simulink model "FlightDataRecorder"  (R2023b)
settings: Solver=VariableStepAuto  StartTime=0.0  StopTime=inf  RelTol=1e-3
libraries: dspindex x28, simulink x4, dspnetwork x4, etargetslib x3, aerolibconvert2 x1
(part 3 of 3)

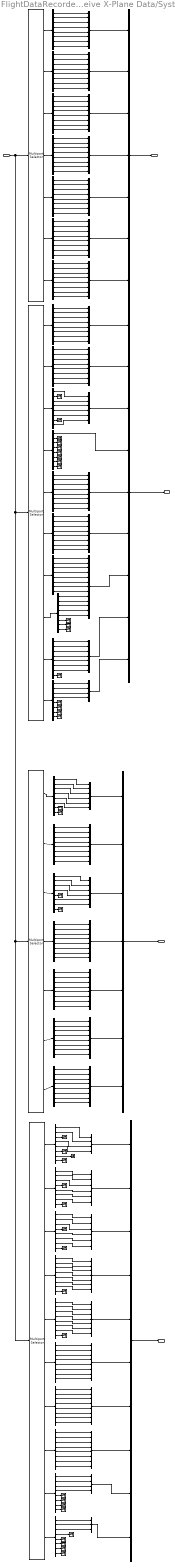
== system FlightDataRecorder/Receive X-Plane Data/Systems ==
  Data : Inport
  Bus Creator{1,3,5..6,11,13..16,18,25..33} (19 alike) : BusCreator  Inputs=8
  Bus Creator{4,10,12,21..22} (5 alike) : BusCreator  Inputs=6
  Bus Creator{8,17,19,23..24} (5 alike) : BusCreator  Inputs=7
  Bus Creator2 : BusCreator  Inputs=9
  Bus Creator20 : BusCreator  Inputs=4
  Bus Creator34 : BusCreator  Inputs=4
  Bus Creator35 : BusCreator  Inputs=3
  Bus Creator36 : BusCreator  Inputs=10
  Bus Creator7 : BusCreator  Inputs=13
  Bus Creator9 : BusCreator  Inputs=4
  Demux{1..34} (34 alike) : Demux  Outputs=8
  Select rows1 : dspindex/Multiport Selector  rowsOrCols=Rows  idxCellArray={107,108,109,110,111,112,113}  idxErrMode=Clip Index
  Select rows2 : dspindex/Multiport Selector  rowsOrCols=Rows  idxCellArray={56,57,58,59,60,61,62}  idxErrMode=Clip Index
  Select rows3 : dspindex/Multiport Selector  rowsOrCols=Rows  idxCellArray={120,121,122,123,124,125,126,127,128,129}  idxErrMode=Clip Index
  Select rows4 : dspindex/Multiport Selector  rowsOrCols=Rows  idxCellArray={97,98,99,100,101,102,103,104,105,106}  idxErrMode=Clip Index
  Terminator{,1..39} (40 alike) : Terminator
  Power systems : Outport
  Operational systems : Outport  Port=2
  Switches : Outport  Port=3
  NAVAID : Outport  Port=4
  wires:
  Demux26/1 -> Bus Creator29/1  "invr 1"
  Bus Creator30/1 -> Bus Creator19/6  "FADEC"
  Demux27/1 -> Bus Creator30/1  "fadec 1"
  Select rows2/6 -> Demux27/1
  Demux27/5 -> Bus Creator30/5  "fadec 5"
  Demux27/3 -> Bus Creator30/3  "fadec 3"
  Demux27/2 -> Bus Creator30/2  "fadec 2"
  Demux27/4 -> Bus Creator30/4  "fadec 4"
  Demux27/6 -> Bus Creator30/6  "fadec 6"
  Demux27/7 -> Bus Creator30/7  "fadec 7"
  Demux27/8 -> Bus Creator30/8  "fadec 8"
  Bus Creator29/1 -> Bus Creator19/5  "Inverter"
  Select rows2/5 -> Demux26/1
  Demux26/5 -> Bus Creator29/5  "invr 5"
  Demux26/3 -> Bus Creator29/3  "invr 3"
  Demux26/2 -> Bus Creator29/2  "invr 2"
  Demux26/4 -> Bus Creator29/4  "invr 4"
  Demux26/6 -> Bus Creator29/6  "invr 6"
  Demux26/7 -> Bus Creator29/7  "invr 7"
  Demux26/8 -> Bus Creator29/8  "invr 8"
  Bus Creator28/1 -> Bus Creator19/4  "Generator"
  Select rows2/4 -> Demux25/1
  Demux25/5 -> Bus Creator28/5  "gen 5"
  Demux25/3 -> Bus Creator28/3  "gen 3"
  Demux25/2 -> Bus Creator28/2  "gen 2"
  Demux25/1 -> Bus Creator28/1  "gen 1"
  Demux25/4 -> Bus Creator28/4  "gen 4"
  Demux25/6 -> Bus Creator28/6  "gen 6"
  Demux25/7 -> Bus Creator28/7  "gen 7"
  Demux25/8 -> Bus Creator28/8  "gen 8"
  Bus Creator27/1 -> Bus Creator19/3  "Battery"
  Select rows2/3 -> Demux24/1
  Demux24/5 -> Bus Creator27/5  "batt 5"
  Demux24/3 -> Bus Creator27/3  "batt 3"
  Demux24/2 -> Bus Creator27/2  "batt 2"
  Demux24/1 -> Bus Creator27/1  "batt 1"
  Demux24/4 -> Bus Creator27/4  "batt 4"
  Demux24/6 -> Bus Creator27/6  "batt 6"
  Demux24/7 -> Bus Creator27/7  "batt 7"
  Demux24/8 -> Bus Creator27/8  "batt 8"
  Demux23/5 -> Bus Creator26/5  "eng idle 5"
  Demux23/3 -> Bus Creator26/3  "eng idle 3"
  Demux23/2 -> Bus Creator26/2  "eng idle 2"
  Demux23/1 -> Bus Creator26/1  "eng idle 1"
  Demux23/4 -> Bus Creator26/4  "eng idle 4"
  Demux23/6 -> Bus Creator26/6  "eng idle 6"
  Bus Creator26/1 -> Bus Creator19/2  "Engine idling"
  Select rows2/2 -> Demux23/1
  Demux23/7 -> Bus Creator26/7  "eng idle 7"
  Demux23/8 -> Bus Creator26/8  "eng idle 8"
  Bus Creator25/1 -> Bus Creator19/1  "Fuel pump"
  Select rows2/1 -> Demux22/1
  Demux22/2 -> Bus Creator25/2  "fuel pump 2"
  Demux22/6 -> Bus Creator25/6  "fuel pump 6"
  Demux22/5 -> Bus Creator25/5  "fuel pump 5"
  Demux22/3 -> Bus Creator25/3  "fuel pump 3"
  Demux22/7 -> Bus Creator25/7  "fuel pump 7"
  Demux22/4 -> Bus Creator25/4  "fuel pump 4"
  Demux22/1 -> Bus Creator25/1  "fuel pump 1"
  Demux22/8 -> Bus Creator25/8  "fuel pump 8"
  Bus Creator18/1 -> Bus Creator19/7  "Ignitier"
  Select rows2/7 -> Demux17/1
  Bus Creator19/1 -> Power systems/1  "Power systems"
  Demux17/2 -> Bus Creator18/2  "igniter 2"
  Demux17/6 -> Bus Creator18/6  "igniter 6"
  Demux17/5 -> Bus Creator18/5  "igniter 5"
  Demux17/3 -> Bus Creator18/3  "igniter 3"
  Demux17/7 -> Bus Creator18/7  "igniter 7"
  Demux17/4 -> Bus Creator18/4  "igniter 4"
  Demux17/1 -> Bus Creator18/1  "igniter 1"
  Demux17/8 -> Bus Creator18/8  "igniter 8"
  Data/1 -> Select rows4/1, Select rows1/1, Select rows3/1, Select rows2/1
  Select rows3/1 -> Demux1/1
  Demux1/2 -> Bus Creator1/2  "pitch"
  Demux1/6 -> Bus Creator1/6  "elevator"
  Demux1/5 -> Bus Creator1/5  "rudder"
  Demux1/3 -> Bus Creator1/3  "R (deg/s)"
  Demux1/7 -> Bus Creator1/7  "speed (knt)"
  Demux1/4 -> Bus Creator1/4  "Q (deg/s)"
  Demux1/1 -> Bus Creator1/1  "heading"
  Demux1/8 -> Bus Creator1/8  "distance (ft)"
  Bus Creator1/1 -> Bus Creator2/1  "Weapon"
  Select rows3/2 -> Demux2/1
  Demux2/2 -> Bus Creator3/2  "vvi cmd"
  Demux2/6 -> Bus Creator3/6  "pressure diff (psi)"
  Demux2/5 -> Bus Creator3/5  "test"
  Demux2/3 -> Bus Creator3/3  "cabin altitude actual"
  Demux2/7 -> Bus Creator3/7  "dump"
  Demux2/4 -> Bus Creator3/4  "vvi actual"
  Demux2/1 -> Bus Creator3/1  "cabin altitude cmd"
  Demux2/8 -> Bus Creator3/8  "bleed"
  Bus Creator3/1 -> Bus Creator2/2  "Pressurisation"
  Select rows3/3 -> Demux3/1
  Demux3/1 -> Bus Creator4/1  "apu equipped"
  Bus Creator4/1 -> Bus Creator2/3  "APU/GPU"
  Demux3/2 -> Terminator/1
  Demux3/3 -> Bus Creator4/2  "apu switch"
  Demux3/4 -> Bus Creator4/3  "apu running"
  Demux3/5 -> Bus Creator4/4  "apu N1"
  Demux3/6 -> Bus Creator4/5  "apu generating"
  Demux3/8 -> Bus Creator4/6  "gpu power"
  Demux3/7 -> Terminator1/1
  Select rows3/4 -> Demux4/1
  Demux4/2 -> Terminator2/1
  Demux4/3 -> Terminator3/1
  Demux4/4 -> Terminator4/1
  Demux4/5 -> Terminator5/1
  Demux4/6 -> Terminator6/1
  Demux4/7 -> Terminator7/1
  Demux4/8 -> Terminator8/1
  Demux4/1 -> Bus Creator2/4  "Radar target"
  Select rows3/5 -> Demux5/1
  Demux5/2 -> Bus Creator5/2  "pump 2a"
  Demux5/6 -> Bus Creator5/6  "fluid 2"
  Demux5/5 -> Bus Creator5/5  "fluid 1"
  Demux5/3 -> Bus Creator5/3  "pump 1b"
  Demux5/7 -> Bus Creator5/7  "pressure 1"
  Demux5/4 -> Bus Creator5/4  "pump 2b"
  Bus Creator5/1 -> Bus Creator2/5  "Hydraulics"
  Demux5/8 -> Bus Creator5/8  "pressure 2"
  Demux5/1 -> Bus Creator5/1  "pump 1a"
  Select rows3/6 -> Demux6/1
  Demux6/2 -> Bus Creator6/2  "bus current 2"
  Demux6/6 -> Bus Creator6/6  "solar output (W)"
  Demux6/5 -> Bus Creator6/5  "eng input (W)"
  Demux6/3 -> Bus Creator6/3  "bus volt 1"
  Demux6/7 -> Bus Creator6/7  "batt capacity (W-hr)"
  Demux6/4 -> Bus Creator6/4  "bus volt 2"
  Demux6/8 -> Bus Creator6/8  "cross"
  Demux6/1 -> Bus Creator6/1  "bus current 1"
  Bus Creator6/1 -> Bus Creator2/6  "Electrical and Solar"
  Select rows3/7 -> Demux7/1
  Demux7/2 -> Bus Creator7/2  "inlet 2"
  Demux7/6 -> Bus Creator7/6  "pitot 2"
  Demux7/5 -> Bus Creator7/5  "pitot 1"
  Demux7/3 -> Bus Creator7/3  "propeller 1"
  Demux7/7 -> Bus Creator7/7  "static 1"
  Demux7/4 -> Bus Creator7/4  "propeller 2"
  Demux7/8 -> Bus Creator7/8  "static 2"
  Demux7/1 -> Bus Creator7/1  "inlet 1"
  Select rows3/8 -> Demux8/1
  Demux8/6 -> Terminator9/1
  Demux8/7 -> Terminator10/1
  Demux8/8 -> Terminator11/1
  Demux8/2 -> Bus Creator7/10  "aoa 2"
  Demux8/5 -> Bus Creator7/13  "window"
  Demux8/3 -> Bus Creator7/11  "left wing"
  Demux8/1 -> Bus Creator7/9  "aoa 1"
  Demux8/4 -> Bus Creator7/12  "right wing"
  Bus Creator7/1 -> Bus Creator2/7  "Icing"
  Select rows3/9 -> Demux9/1
  Demux9/2 -> Bus Creator8/2  "caut time"
  Demux9/6 -> Bus Creator8/6  "gear warning"
  Demux9/5 -> Bus Creator8/5  "gear work"
  Demux9/3 -> Bus Creator8/3  "warning work"
  Demux9/7 -> Bus Creator8/7  "stall warning"
  Demux9/4 -> Bus Creator8/4  "caut work"
  Demux9/1 -> Bus Creator8/1  "warning time"
  Bus Creator8/1 -> Bus Creator2/8  "Warnings"
  Demux9/8 -> Terminator12/1
  Select rows3/10 -> Demux10/1
  Demux10/1 -> Bus Creator9/1  "leg time"
  Demux10/2 -> Bus Creator9/2  "leg type"
  Demux10/3 -> Bus Creator9/3  "leg latitude"
  Demux10/4 -> Bus Creator9/4  "leg longitude"
  Demux10/5 -> Terminator13/1
  Demux10/6 -> Terminator14/1
  Demux10/7 -> Terminator15/1
  Demux10/8 -> Terminator16/1
  Bus Creator9/1 -> Bus Creator2/9  "Flight plan legs"
  Bus Creator2/1 -> Operational systems/1  "Operational systems"
  Select rows1/1 -> Demux11/1
  Demux11/2 -> Bus Creator10/2  "NAV lights"
  Demux11/6 -> Bus Creator10/6  "Taxi lights"
  Demux11/5 -> Bus Creator10/5  "Landing lights"
  Demux11/3 -> Bus Creator10/3  "Beacon lights"
  Demux11/4 -> Bus Creator10/4  "Strobe lights"
  Demux11/1 -> Bus Creator10/1  "AVIO"
  Demux11/8 -> Terminator17/1
  Demux11/7 -> Terminator18/1
  Bus Creator10/1 -> Bus Creator17/1  "Light switches"
  Demux12/2 -> Bus Creator11/2  "EFIS 1"
  Demux12/6 -> Bus Creator11/6  "HSI arc"
  Demux12/5 -> Bus Creator11/5  "HSI 2"
  Demux12/3 -> Bus Creator11/3  "EFIS 2"
  Demux12/4 -> Bus Creator11/4  "HSI 1"
  Demux12/1 -> Bus Creator11/1  "ECAM"
  Demux12/8 -> Bus Creator11/8  "map range"
  Demux12/7 -> Bus Creator11/7  "map"
  Select rows1/2 -> Demux12/1
  Bus Creator11/1 -> Bus Creator17/2  "EFIS"
  Select rows1/3 -> Demux13/1
  Bus Creator12/1 -> Bus Creator17/3  "AP/FDIR/HUD"
  Demux13/5 -> Terminator19/1
  Demux13/8 -> Terminator20/1
  Demux14/2 -> Bus Creator13/2  "inlet"
  Demux14/6 -> Bus Creator13/6  "pitot 2"
  Demux14/5 -> Bus Creator13/5  "pitot 1"
  Demux14/3 -> Bus Creator13/3  "propeller"
  Demux14/4 -> Bus Creator13/4  "windows"
  Demux14/1 -> Bus Creator13/1  "all"
  Demux14/8 -> Bus Creator13/8  "wing"
  Demux14/7 -> Bus Creator13/7  "AOA"
  Select rows1/4 -> Demux14/1
  Bus Creator13/1 -> Bus Creator17/4  "Anti-ice"
  Demux15/2 -> Bus Creator14/2  "air 2"
  Demux15/6 -> Bus Creator14/6  "manual ignition 2"
  Demux15/5 -> Bus Creator14/5  "manual ignition 1"
  Demux15/3 -> Bus Creator14/3  "auto ignition 1"
  Demux15/4 -> Bus Creator14/4  "auto ignition 2"
  Demux15/1 -> Bus Creator14/1  "air 1"
  Demux15/8 -> Bus Creator14/8  "right tank"
  Demux15/7 -> Bus Creator14/7  "left tank"
  Select rows1/5 -> Demux15/1
  Bus Creator14/1 -> Bus Creator17/5  "Fuel"
  Demux16/2 -> Bus Creator15/2  "prepro 2"
  Demux16/6 -> Bus Creator15/6  "SAS roll"
  Demux16/5 -> Bus Creator15/5  "SAS pitch"
  Demux16/3 -> Bus Creator15/3  "clutch 1"
  Demux16/4 -> Bus Creator15/4  "clutch 2"
  Demux16/1 -> Bus Creator15/1  "prepro 1"
  Demux16/8 -> Bus Creator15/8  "auto brake"
  Demux16/7 -> Bus Creator15/7  "SAS yaw"
  Select rows1/6 -> Demux16/1
  Bus Creator15/1 -> Bus Creator17/6  "Clutch/SAS"
  Demux18/2 -> Bus Creator16/2  "radal (ft)"
  Demux18/6 -> Bus Creator16/6  "water scoop"
  Demux18/5 -> Bus Creator16/5  "puffr"
  Demux18/3 -> Bus Creator16/3  "propeller"
  Demux18/4 -> Bus Creator16/4  "feathering mode"
  Demux18/1 -> Bus Creator16/1  "total energy"
  Demux18/8 -> Bus Creator16/8  "chute"
  Demux18/7 -> Bus Creator16/7  "arrester hook"
  Select rows1/7 -> Demux18/1
  Bus Creator16/1 -> Bus Creator17/7  "Miscellaneous"
  Demux13/7 -> Bus Creator12/6  "HUD brightness"
  Demux13/6 -> Bus Creator12/5  "HUD power"
  Demux13/4 -> Bus Creator12/4  "FDIR roll cmd"
  Demux13/2 -> Bus Creator12/2  "FDIR mode"
  Demux13/1 -> Bus Creator12/1  "AP"
  Demux13/3 -> Bus Creator12/3  "FDIR pitch cmd"
  Bus Creator17/1 -> Switches/1  "Switches"
  Bus Creator20/1 -> Bus Creator36/1  "COM 1/2 frequency"
  Bus Creator21/1 -> Bus Creator36/2  "NAV 1/2 frequency"
  Demux19/3 -> Terminator21/1
  Demux19/6 -> Terminator22/1
  Demux19/1 -> Bus Creator20/1  "COM 1"
  Demux19/2 -> Bus Creator20/2  "COM 1 standby"
  Demux19/4 -> Bus Creator20/3  "COM 2"
  Demux19/5 -> Bus Creator20/4  "COM 2 standby"
  Demux19/7 -> Terminator23/1  "transit status"
  Demux19/8 -> Terminator24/1
  Demux20/4 -> Terminator25/1
  Demux20/8 -> Terminator26/1
  Demux20/1 -> Bus Creator21/1  "NAV 1"
  Demux20/5 -> Bus Creator21/4  "NAV 2"
  Demux20/2 -> Bus Creator21/2  "NAV 1 standby"
  Demux20/6 -> Bus Creator21/5  "NAV 2 standby"
  Demux20/3 -> Bus Creator21/3  "NAV 1 type"
  Demux20/7 -> Bus Creator21/6  "NAV 2 type"
  Select rows4/2 -> Demux20/1
  Select rows4/1 -> Demux19/1
  Bus Creator22/1 -> Bus Creator36/3  "NAV 1/2 OBS"
  Demux21/4 -> Terminator27/1
  Demux21/8 -> Terminator28/1
  Demux21/1 -> Bus Creator22/1  "NAV 1 OBS"
  Demux21/5 -> Bus Creator22/4  "NAV 2 OBS"
  Demux21/2 -> Bus Creator22/2  "NAV 1 s-crs"
  Demux21/6 -> Bus Creator22/5  "NAV 2 s-crs"
  Demux21/3 -> Bus Creator22/3  "NAV 1 flag"
  Demux21/7 -> Bus Creator22/6  "NAV 2 flag"
  Select rows4/3 -> Demux21/1
  Bus Creator23/1 -> Bus Creator36/4  "NAV 1 deflections"
  Demux28/8 -> Terminator30/1
  Select rows4/4 -> Demux28/1
  Demux28/6 -> Bus Creator23/6  "NAV 1 h-def"
  Demux28/1 -> Bus Creator23/1  "NAV 1 n-type"
  Demux28/4 -> Bus Creator23/4  "NAV 1 r-brg"
  Demux28/2 -> Bus Creator23/2  "NAV 1 to-fr"
  Demux28/3 -> Bus Creator23/3  "NAV 1 m-crs"
  Demux28/5 -> Bus Creator23/5  "NAV 1 dme-d"
  Demux28/7 -> Bus Creator23/7  "NAV 1 v-def"
  Bus Creator24/1 -> Bus Creator36/5  "NAV 2 deflections"
  Demux29/8 -> Terminator29/1
  Select rows4/5 -> Demux29/1
  Demux29/6 -> Bus Creator24/6  "NAV 2 h-def"
  Demux29/4 -> Bus Creator24/4  "NAV 2 r-brg"
  Demux29/2 -> Bus Creator24/2  "NAV 2 to-fr"
  Demux29/3 -> Bus Creator24/3  "NAV 2 m-crs"
  Demux29/5 -> Bus Creator24/5  "NAV 2 dme-d"
  Demux29/7 -> Bus Creator24/7  "NAV 2 v-def"
  Demux29/1 -> Bus Creator24/1  "NAV 2 n-type"
  Bus Creator31/1 -> Bus Creator36/6  "ADF 1/2"
  Demux30/8 -> Bus Creator31/8  "ADF 2 n-type"
  Select rows4/6 -> Demux30/1
  Demux30/6 -> Bus Creator31/6  "ADF 2 card"
  Demux30/4 -> Bus Creator31/4  "ADF 1 n-type"
  Demux30/2 -> Bus Creator31/2  "ADF 1 card"
  Demux30/3 -> Bus Creator31/3  "ADF 1 r-brg"
  Demux30/5 -> Bus Creator31/5  "ADF 2 freq"
  Demux30/7 -> Bus Creator31/7  "ADF 2 r-brg"
  Demux30/1 -> Bus Creator31/1  "ADF 1 freq"
  Bus Creator32/1 -> Bus Creator36/7  "DME"
  Demux31/8 -> Bus Creator32/8  "DME-3 frequency"
  Demux31/6 -> Bus Creator32/6  "DME time"
  Demux31/4 -> Bus Creator32/4  "DME distance"
  Demux31/2 -> Bus Creator32/2  "DME mode"
  Demux31/3 -> Bus Creator32/3  "DME found"
  Demux31/5 -> Bus Creator32/5  "DME speed"
  Demux31/7 -> Bus Creator32/7  "DME n-type"
  Select rows4/7 -> Demux31/1
  Demux31/1 -> Bus Creator32/1  "DME"
  Bus Creator33/1 -> Bus Creator36/8  "GPS"
  Demux32/8 -> Bus Creator33/8  "vdef dots"
  Demux32/6 -> Bus Creator33/6  "rel bearing"
  Demux32/4 -> Bus Creator33/4  "OBS (mag)"
  Demux32/2 -> Bus Creator33/2  "GPS index"
  Demux32/3 -> Bus Creator33/3  "distance (nmi)"
  Demux32/5 -> Bus Creator33/5  "crs (mag)"
  Demux32/7 -> Bus Creator33/7  "hdef dots"
  Select rows4/8 -> Demux32/1
  Demux32/1 -> Bus Creator33/1  "GPS mode"
  Bus Creator34/1 -> Bus Creator36/9  "XPNDR"
  Select rows4/9 -> Demux33/1
  Demux33/5 -> Terminator31/1
  Demux33/8 -> Terminator34/1
  Demux33/7 -> Terminator33/1
  Demux33/6 -> Terminator32/1
  Demux33/1 -> Bus Creator34/1  "transponder mode"
  Demux33/2 -> Bus Creator34/2  "transponder set"
  Demux33/3 -> Bus Creator34/3  "transponder ID"
  Demux33/4 -> Bus Creator34/4  "transponder inter"
  Bus Creator35/1 -> Bus Creator36/10  "MARKER"
  Select rows4/10 -> Demux34/1
  Demux34/5 -> Terminator35/1
  Demux34/8 -> Terminator38/1
  Demux34/7 -> Terminator37/1
  Demux34/6 -> Terminator36/1
  Demux34/1 -> Bus Creator35/1  "outer marker signal"
  Demux34/2 -> Bus Creator35/2  "middle marker signal"
  Demux34/3 -> Bus Creator35/3  "inner marker signal"
  Demux34/4 -> Terminator39/1  "audio active"
  Bus Creator36/1 -> NAVAID/1  "NAVAID"

== system FlightDataRecorder/Receive X-Plane Data/Thrust vectoring ==
  Data : Inport
  Bus Creator1 : BusCreator  Inputs=8
  Bus Creator3 : BusCreator  Inputs=8
  Demux1 : Demux  Outputs=8
  Demux11 : Demux  Outputs=8
  Select rows1 : dspindex/Multiport Selector  rowsOrCols=Rows  idxCellArray={79,80}  idxErrMode=Clip Index
  Vertical : Outport
  Lateral : Outport  Port=2
  wires:
  Demux1/7 -> Bus Creator1/7  "lateral thrust 7"
  Demux1/8 -> Bus Creator1/8  "lateral thrust 8"
  Demux1/6 -> Bus Creator1/6  "lateral thrust 6"
  Demux1/5 -> Bus Creator1/5  "lateral thrust 5"
  Demux1/1 -> Bus Creator1/1  "lateral thrust 1"
  Demux1/2 -> Bus Creator1/2  "lateral thrust 2"
  Demux1/3 -> Bus Creator1/3  "lateral thrust 3"
  Demux1/4 -> Bus Creator1/4  "lateral thrust 4"
  Select rows1/2 -> Demux1/1
  Demux11/7 -> Bus Creator3/7  "vertical thrust 7"
  Demux11/8 -> Bus Creator3/8  "vertical thrust 8"
  Demux11/6 -> Bus Creator3/6  "vertical thrust 6"
  Demux11/5 -> Bus Creator3/5  "vertical thrust 5"
  Demux11/1 -> Bus Creator3/1  "vertical thrust 1"
  Demux11/2 -> Bus Creator3/2  "vertical thrust 2"
  Demux11/3 -> Bus Creator3/3  "vertical thrust 3"
  Demux11/4 -> Bus Creator3/4  "vertical thrust 4"
  Data/1 -> Select rows1/1
  Select rows1/1 -> Demux11/1
  Bus Creator3/1 -> Vertical/1  "Vertical thrusters"
  Bus Creator1/1 -> Lateral/1  "Lateral thrusters"

== system FlightDataRecorder/Receive X-Plane Data/Time ==
  note: Zulu (GMT) time is in decimal hours (e.g. 3.5 is 3:30 am)
  Data : Inport
  Bus Creator : BusCreator  Inputs=5
  Demux : Demux  Outputs=8
  Select rows : dspindex/Multiport Selector  rowsOrCols=Rows  idxCellArray={2}  idxErrMode=Clip Index
  Terminator : Terminator
  Terminator1 : Terminator
  Terminator2 : Terminator
  Time : Outport
  wires:
  Select rows/1 -> Demux/1
  Bus Creator/1 -> Time/1  "Time"
  Data/1 -> Select rows/1
  Demux/1 -> Terminator/1  "real"
  Demux/4 -> Terminator1/1  "timer"
  Demux/5 -> Terminator2/1
  Demux/2 -> Bus Creator/1  "total time"
  Demux/3 -> Bus Creator/2  "mission time"
  Demux/6 -> Bus Creator/3  "zulu (GMT)"
  Demux/7 -> Bus Creator/4  "local"
  Demux/8 -> Bus Creator/5  "hobbs"

== system FlightDataRecorder/Receive X-Plane Data/Weights ==
  note: CG position is measured
      | aft of reference point (ft)
  Data : Inport
  Bus Creator10 : BusCreator  Inputs=8
  Bus Creator12 : BusCreator  Inputs=6
  Demux11 : Demux  Outputs=8
  Demux12 : Demux  Outputs=8
  Select rows1 : dspindex/Multiport Selector  rowsOrCols=Rows  idxCellArray={63,64}  idxErrMode=Clip Index
  Terminator1 : Terminator
  Aircraft weights : Outport
  Fuel weights : Outport  Port=2
  CG : Outport  Port=3
  wires:
  Data/1 -> Select rows1/1
  Select rows1/1 -> Demux11/1
  Bus Creator10/1 -> Fuel weights/1  "Fuel weights"
  Demux11/1 -> Bus Creator10/1  "fuel tank 1"
  Demux11/2 -> Bus Creator10/2  "fuel tank 2"
  Demux11/3 -> Bus Creator10/3  "fuel tank 3"
  Demux11/5 -> Bus Creator10/5  "fuel tank 5"
  Demux11/8 -> Bus Creator10/8  "fuel tank 8"
  Demux11/6 -> Bus Creator10/6  "fuel tank 6"
  Demux11/4 -> Bus Creator10/4  "fuel tank 4"
  Demux11/7 -> Bus Creator10/7  "fuel tank 7"
  Select rows1/2 -> Demux12/1
  Bus Creator12/1 -> Aircraft weights/1  "Weights (lb)"
  Demux12/1 -> Bus Creator12/1  "empty"
  Demux12/2 -> Bus Creator12/2  "payload"
  Demux12/3 -> Bus Creator12/3  "fuel"
  Demux12/5 -> Bus Creator12/5  "current"
  Demux12/6 -> Bus Creator12/6  "maximum"
  Demux12/4 -> Bus Creator12/4  "jettisonable"
  Demux12/7 -> Terminator1/1
  Demux12/8 -> CG/1  "CG position (ft)"

== matlab function FlightDataRecorder/Receive X-Plane Data/Set data/Package data string ==
  data: y1 output; u input; y2 output
function [y1,y2] = fcn(u)
%#codegen
y1 = uint8('DSEL0');
y2 = uint32(u);

== matlab function FlightDataRecorder/Receive X-Plane Data/Set data/Unselect frame rate <0> ==
  data: y1 output; y2 output
function [y1,y2] = fcn()
%#codegen
y1 = uint8('USEL0');
y2 = uint32(0);

== matlab function FlightDataRecorder/Receive X-Plane Data/Data parser ==
  data: msg input; Data output single size=[134 8]; Length input
function Data = msgParser(msg,Length)
% MSG:    UDP data string
% LENGTH: byte length of msg

% Paser code adapted from work by M A Zahana (2014). See
% https://uk.mathworks.com/matlabcentral/fileexchange/47144-simulink-xplane10-communication-via-udp

DataLength = Length-5; % Length of data stream minus message prologue (DATA@)
Byte       = 6; % First byte to start collecting data
Packets    = DataLength/36; % Number of data packets (each is 36 bytes long)
MaxPackets = 134;
Params     = 8; % Number of parameters in each data packet

% Initilalise DATA
% Rows: Index, Columns: Parameters
Data = single(zeros(MaxPackets,Params));

for i = 1:Length
    % Find start of message prologue (just in case!)
    if char(msg(i)) == 'D' && char(msg(i+1)) == 'A'  
        for j = 1:Packets
            % Get packet index
            idx = single(msg(Byte));

            % Extract parameters from each 4-byte sequence
            % Note: need to add 1 to idx in case <frame rate> group is
            % added (accidently since it is never called from this block,
            % or if it is set on start-up; it has an idx of 0, hence will
            % crash Simulink)
            Byte = Byte + 4;
            Data(idx+1,1) = typecast(msg(Byte:Byte+3),'single');
            Byte = Byte + 4;
            Data(idx+1,2) = typecast(msg(Byte:Byte+3),'single');
            Byte = Byte + 4;
            Data(idx+1,3) = typecast(msg(Byte:Byte+3),'single');
            Byte = Byte + 4;
            Data(idx+1,4) = typecast(msg(Byte:Byte+3),'single');
            Byte = Byte + 4;
            Data(idx+1,5) = typecast(msg(Byte:Byte+3),'single');
            Byte = Byte + 4;
            Data(idx+1,6) = typecast(msg(Byte:Byte+3),'single');
            Byte = Byte + 4;
            Data(idx+1,7) = typecast(msg(Byte:Byte+3),'single');
            Byte = Byte + 4;
            Data(idx+1,8) = typecast(msg(Byte:Byte+3),'single');
            
            % Increment BYTE for next packet on next loop
            Byte = Byte + 4;
        end
        break
    end
end

== matlab function FlightDataRecorder/Receive X-Plane Data/Deselect all data in first instance/Unselect all data ==
  data: y1 output; y2 output
function [y1,y2] = fcn()
%#codegen
y1 = uint8('USEL0');
y2 = uint32(1:133);
% Can't deselect entire range since causes error, so leave <0>
